simulink model "inflowmodel"  (R2024a)
settings: Solver=VariableStepAuto  StartTime=0.0  StopTime=10.0  RelTol=1e-3
settings Model: Creator=10335  LastModifiedBy=10335

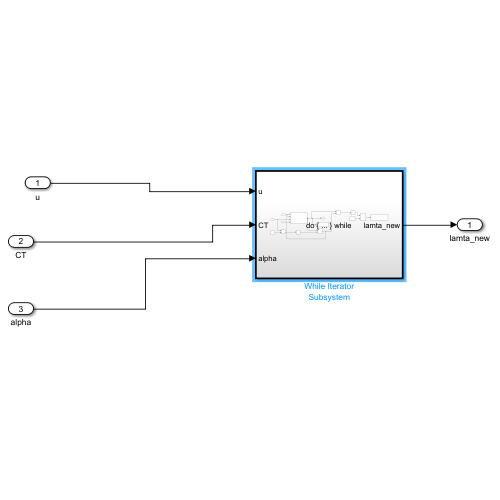
[thumbnail: Simulink's stored preview of the top-level diagram]
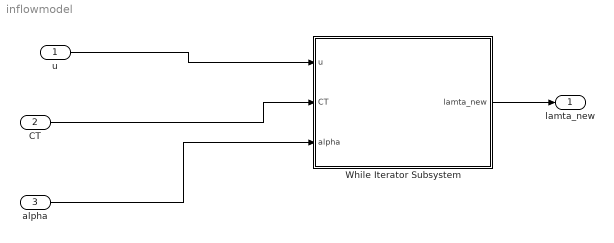
== system inflowmodel ==
  u : Inport
  CT : Inport  Port=2
  alpha : Inport  Port=3
  While Iterator Subsystem : Subsystem  TreatAsAtomicUnit=on
  lamta_new : Outport
  wires:
  CT/1 -> While Iterator Subsystem/2(CT)
  While Iterator Subsystem/1(lamta_new) -> lamta_new/1
  alpha/1 -> While Iterator Subsystem/3(alpha)
  u/1 -> While Iterator Subsystem/1(u)

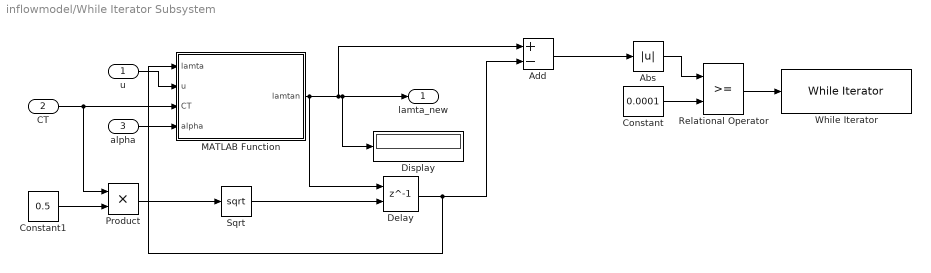
== system inflowmodel/While Iterator Subsystem ==
  u : Inport
  CT : Inport  Port=2
  alpha : Inport  Port=3
  Abs : Abs  SaturateOnIntegerOverflow=off
  Add : Sum  Inputs=+-
  Constant : Constant  Value=0.0001
  Constant1 : Constant  Value=0.5
  Delay : Delay  DelayLength=1  InitialConditionSource=Input port
      settings: InputPortMap=u0,p4
  Display : Display
  MATLAB Function : MATLAB Function  TreatAsAtomicUnit=on
  Product : Product
  Relational Operator : RelationalOperator  OutDataTypeStr=boolean  RndMeth=Simplest  InputSameDT=off
  Sqrt : Sqrt
  While Iterator : WhileIterator  MaxIters=8  WhileBlockType=do-while
  lamta_new : Outport
  wires:
  Delay/1 -> Add/2, MATLAB Function/1(lamta)
  Sqrt/1 -> Delay/2
  Abs/1 -> Relational Operator/1
  CT/1 -> MATLAB Function/3(CT), Product/1
  Constant1/1 -> Product/2
  MATLAB Function/1(lamtan) -> lamta_new/1, Display/1, Add/1, Delay/1
  u/1 -> MATLAB Function/2(u)
  Constant/1 -> Relational Operator/2
  alpha/1 -> MATLAB Function/4(alpha)
  Product/1 -> Sqrt/1
  Add/1 -> Abs/1
  Relational Operator/1 -> While Iterator/1

== matlab function inflowmodel/While Iterator Subsystem/MATLAB Function ==
  data: lamta input; u input; lamtan output; CT input; alpha input
function lamtan = fcn( lamta,u,CT,alpha)

alpha=alpha/57.3;
f=lamta-u*tan(alpha)-0.5*CT/sqrt(lamta^2+u^2);
df=1+lamta*CT/2*power(u^2+lamta^2,-1.5);

lamtan=lamta-f/df;
